simulink library "adcUtils"  (R2023b)
settings: Solver=ode45  StartTime=0.0  StopTime=10.0  RelTol=1e-3  EnableMultiTasking=on
undefined symbols (not defined in the file): angle_sensor_range, Ts, uint_range_10bit
libraries: $bdroot x1
settings Model: Creator=jrivitus  LastModifiedBy=ykajita
settings SolverCC: AlgebraicLoopSolver=TrustRegion
settings DataIOCC: LimitDataPoints=on  SaveFormat=Array  ReturnWorkspaceOutputs=off
settings OptimizationCC: ExpressionDepthLimit=2147483647  LifeSpan=inf
settings DebuggingCC: SolverPrmCheckMsg=warning  ParameterPrecisionLossMsg=none  FcnCallInpInsideContextMsg=warning  UnconnectedInputMsg=warning  UnconnectedOutputMsg=warning  UnconnectedLineMsg=warning  StateNameClashWarn=warning  PregeneratedLibrarySubsystemCodeDiagnostic=none  SFUnexpectedBacktrackingDiag=warning  SFNoUnconditionalDefaultTransitionDiag=warning  SFExecutionAtInitializationDiag=none  ArithmeticOperatorsInVariantConditions=warning
settings HardwareCC: ProdBitPerPointer=32  ProdBitPerSizeT=32  ProdBitPerPtrDiffT=32  ProdLargestAtomicFloat=None  ProdIntDivRoundTo=Undefined  ProdEndianess=Unspecified  ProdWordSize=32  ProdHWDeviceType=32-bit Generic
settings ModelReferenceCC: EnableRefExpFcnMdlSchedulingChecks=on  PropagateSignalLabelsOutOfModel=off
settings SFSimCC: SimUseLocalCustomCode=off
settings RTWCC: RTWUseLocalCustomCode=off  DLArmComputeVersion=19.05
settings CodeAppCC: StateflowObjectComments=on
settings GRTTargetCC: TargetLangStandard=C89/C90 (ANSI)  CombineOutputUpdateFcns=off  GRTInterface=on
settings ConfigComp: CovMetricSettings=dw  CovSaveCumulativeToWorkspaceVar=on  CovSaveSingleToWorkspaceVar=on  CovExternalEMLEnable=off  CovSFcnEnable=off

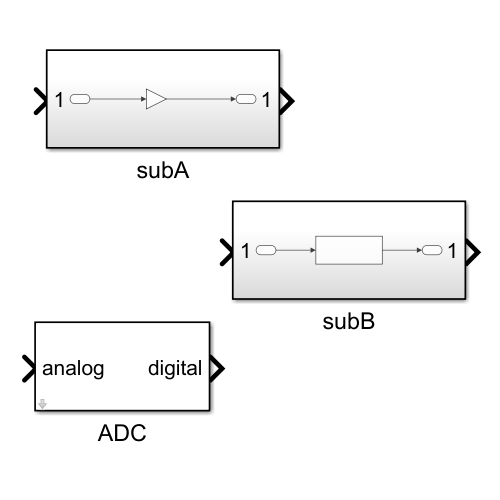
[thumbnail: Simulink's stored preview of the top-level diagram]
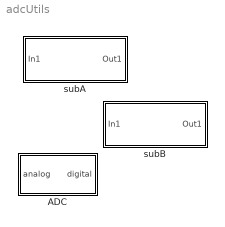
== system adcUtils ==
  ADC : Subsystem  mask{analog_range=angle_sensor_range, digital_range=uint_range_10bit, outputType=uint16, sampleRate=Ts}
      mask prompts: analog_range "Analog range:"; digital_range "Digital range:"; outputType "Output data type:"; sampleRate "Sampling rate:"
  subA : Subsystem
  subB : Subsystem

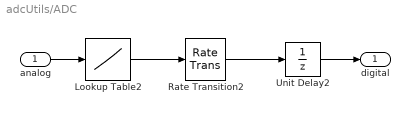
== system adcUtils/ADC ==
  analog : Inport
  Lookup Table2 : Lookup_n-D  NumberOfTableDimensions=1  BreakpointsForDimension1=analog_range  Table=digital_range  ExtrapMethod=Clip  OutDataTypeStr=outputType
      settings: AttributesFormatString=Output data type: %<OutDataTypeStr>
  Rate Transition2 : RateTransition  Integrity=off  OutPortSampleTime=0
  Unit Delay2 : UnitDelay  SampleTime=sampleRate  HasFrameUpgradeWarning=on
  digital : Outport  VectorParamsAs1DForOutWhenUnconnected=off
  wires:
  Unit Delay2/1 -> digital/1
  analog/1 -> Lookup Table2/1
  Rate Transition2/1 -> Unit Delay2/1
  Lookup Table2/1 -> Rate Transition2/1

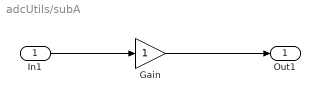
== system adcUtils/subA ==
  In1 : Inport
  Gain : Gain
  Out1 : Outport
  wires:
  In1/1 -> Gain/1
  Gain/1 -> Out1/1

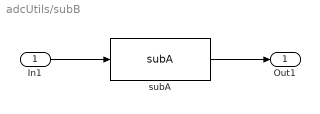
== system adcUtils/subB ==
  In1 : Inport
  subA : $bdroot/subA  SystemSampleTime=-1  VariantActivationTime=update diagram  AllowFlexibleInterface=on  Latency=0  AutoFrameSizeCalculation=off
  Out1 : Outport
  wires:
  subA/1 -> Out1/1
  In1/1 -> subA/1
